simulink library "Steer_Ackermann_Systems"  (R2026a)
settings: Solver=VariableStepAuto
undefined symbols (not defined in the file): Susp
libraries: Steer_Ackermann x2, Steer_Ackermann_WheelsOnly x1, sm_car_lib x1
Description:
  | Component of Simscape Vehicle Templates Library
  | 
  | Copyright 2018-2026 The MathWorks, Inc.
settings Model: Creator=smiller  LastModifiedBy=smiller

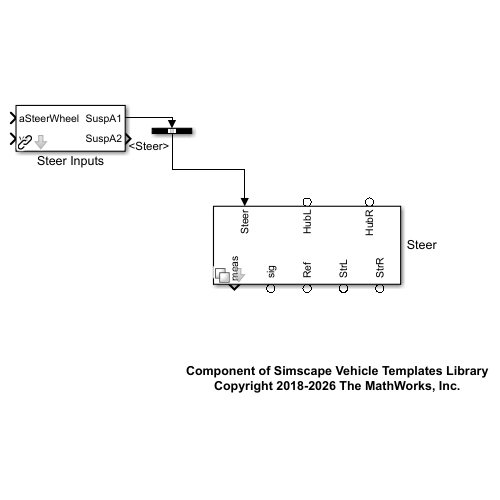
[thumbnail: Simulink's stored preview of the top-level diagram]
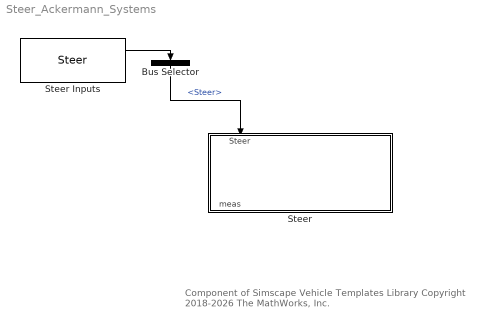
== system Steer_Ackermann_Systems ==
  note: Component of Simscape Vehicle Templates Library
      | Copyright 2018-2026 The MathWorks, Inc.
  Bus Selector : BusSelector  OutputSignals=Steer
  Steer : Subsystem  Variant=on  VariantControl=Variant1  mask{Steer=Susp.Steer, VariantLabel=Susp.Steer.class.Value, InitTriggerDropdown=1}
      mask prompts: Steer "Steer Parameters"; VariantLabel "Variant Label"; InitTriggerDropdown "Initialization Trigger Dropdown"
      mask init:
      | curblk = gcb;
      | 
      | % Set variant for this subsystem
      | set_param(curblk,'LabelModeActiveChoice',VariantLabel);
      | 
      | % Trigger Mask Initialization for 
      | % variant subsystems below this level
      | sm_car_lib_maskInitTrigger(curblk)
      | 
      | %% Find other blocks to trigger
      | %f=Simulink.FindOptions('FollowLinks',1,'RegExp',1);
      | %h=Simulink.findBlocks(curblk,'InitTriggerDropdown','.*',f);
      | 
      | %% Trigger mask initialization
      | %for i=1:length(h)
      | %    try % Avoid setting parameter within library links
      | %        set_param(h(i),'InitTriggerDropdown',get_param(curblk,'InitTriggerDropdown'));
      | 
      | % For debugging
      | %        disp([curblk ': Success for ' getfullname(h(i))]);
      | %    catch
      | %        disp([curblk ': Failed for ' getfullname(h(i))]);
      | 
      | %    end
      | %end
      settings: AttributesFormatString=%<ActiveVariant>
      mask TypeOptions InitTriggerDropdown: 0 | 1
      mask Display: disp(' ')
  Steer Inputs : sm_car_lib/Control/Steer  Steer=Control.Default.Steer
  wires:
  Steer Inputs/1 -> Bus Selector/1
  Bus Selector/1 -> Steer/1(Steer)  "<Steer>"

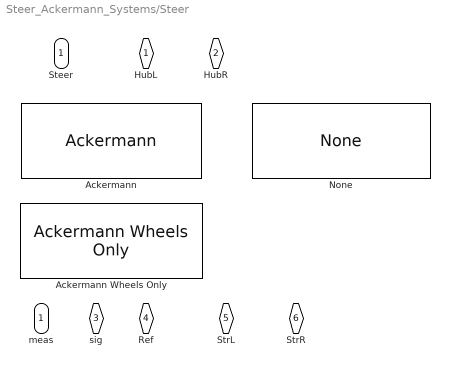
== system Steer_Ackermann_Systems/Steer ==
  Steer : Inport
  Ackermann : Steer_Ackermann/Ackermann  VariantControl=Ackermann  InitTriggerDropdown=1  hp_wheel=Steer.Wheel.sMount.Value  wheel_axis_incl=Steer.Wheel.aAxis.Value  Wheel=Steer.Wheel  whl2rack_filter=1/Steer.Rack.fActuatorCutoff.Value  yTrack=Steer.xTrack.Value  xwheelbase=Steer.xWheelbase.Value  steer_ratio=Susp.Steer.rSteer.Value  clr_wheel=Visual.SteeringWheel.clr  opc_wheel=Visual.part.opc  DriverHuman=Steer.DriverHuman
  Ackermann Wheels Only : Steer_Ackermann_WheelsOnly/Ackermann Wheels Only  VariantControl=AckermannWheelsOnly  InitTriggerDropdown=0  whl2rack_filter=1/Steer.Rack.fActuatorCutoff.Value  yTrack=Steer.xTrack.Value  xwheelbase=Steer.xWheelbase.Value  steer_ratio=Susp.Steer.rSteer.Value
  None : Steer_Ackermann/None  SystemSampleTime=-1  VariantControl=None  VariantActivationTime=update diagram  EmptyChoice=off  PassThrough=off  PassThroughVariantControl=(default)  EmptyChoiceVariantControl=(default)  AllowFlexibleInterface=on  Latency=0  AutoFrameSizeCalculation=off
  " HubL" : PMIOPort  Side=Left
  " HubR" : PMIOPort  Port=2  Side=Left
  " sig" : PMIOPort  Port=3  Side=Right
  " Ref" : PMIOPort  Port=4  Side=Right
  " StrL" : PMIOPort  Port=5  Side=Right
  " StrR" : PMIOPort  Port=6  Side=Right
  meas : Outport  VectorParamsAs1DForOutWhenUnconnected=off
